simulink model "corrip"  (Simulink 3.00)
settings: Solver=ode5  SolverMode=SingleTasking  StartTime=0.0  StopTime=2.335  FixedStep=0.001  MaxStep=0.001  RelTol=1e-3  AbsTol=1e-3
values from neighbouring files (symbols this model uses):
  b = 5E-5    (= 5e-05)    [Constants.m]
  J = 1    [Constants.m]
  Ka = 20    [Constants.m]
  Km = 1.36    [Constants.m]
  Kp = 50    [Constants.m]
settings Model: SaveTime=off  SaveOutput=off

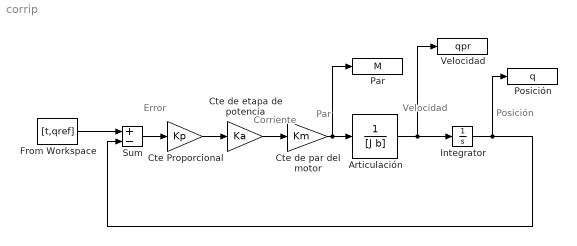
== system corrip ==
  note: Corriente
  note: Error
  note: Velocidad
  note: Posición
  note: Par
  Articulación : TransferFcn  Numerator=[1]  Denominator=[J b]
  Cte Proporcional : Gain  Gain=Kp  SaturateOnIntegerOverflow=on
  Cte de etapa de potencia : Gain  Gain=Ka  SaturateOnIntegerOverflow=on
  Cte de par del motor : Gain  Gain=Km  SaturateOnIntegerOverflow=on
  From Workspace : FromWorkspace  VariableName=[t,qref]  SampleTime=0.001  HoldFinalValue=off
  Integrator : Integrator  ExternalReset=none  InitialConditionSource=internal  InitialCondition=0  LimitOutput=off  UpperSaturationLimit=inf  LowerSaturationLimit=-inf  ShowSaturationPort=off  ShowStatePort=off  AbsoluteTolerance=auto
  Par : ToWorkspace  VariableName=M  SampleTime=0  SaveFormat=Matrix
      settings: Buffer=2335
  Posición : ToWorkspace  VariableName=q  SampleTime=0  SaveFormat=Matrix
      settings: Buffer=2335
  Sum : Sum  Inputs=+-  SaturateOnIntegerOverflow=on
  Velocidad : ToWorkspace  VariableName=qpr  SampleTime=0  SaveFormat=Matrix
      settings: Buffer=2335
  wires:
  Cte de etapa de potencia/1 -> Cte de par del motor/1
  From Workspace/1 -> Sum/1
  Cte Proporcional/1 -> Cte de etapa de potencia/1
  Sum/1 -> Cte Proporcional/1
  Cte de par del motor/1 -> Articulación/1, Par/1
  Articulación/1 -> Integrator/1, Velocidad/1
  Integrator/1 -> Sum/2, Posición/1
